simulink subsystem "PathFollowingController"  (R2022a)
settings: Solver=VariableStepAuto  StartTime=0.0  StopTime=10.0  RelTol=1e-3
undefined symbols (not defined in the file): constr, DE2019, DiscIntNeverNeededParam, ENVMT, Lbooth, loiterStates, params
libraries: simulink x16, dspsigops x1
(part 1 of 2)
settings Model: Creator=dylaneijkelhof  LastModifiedBy=kebl6571
settings SolverCC: AlgebraicLoopSolver=TrustRegion
settings DebuggingCC: UnconnectedInputMsg=warning  UnconnectedOutputMsg=warning  UnconnectedLineMsg=warning  SFMachineParentedDataDiag=warning

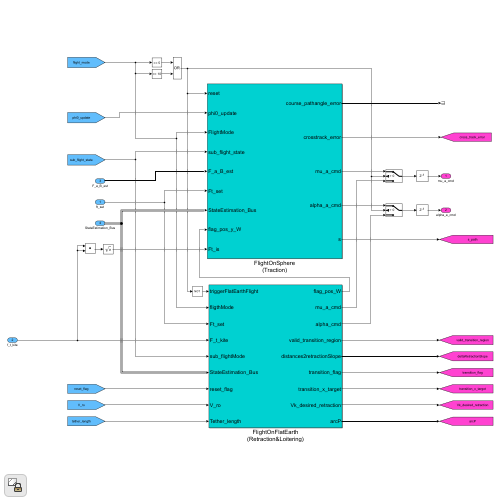
[thumbnail: Simulink's stored preview of the top-level diagram]
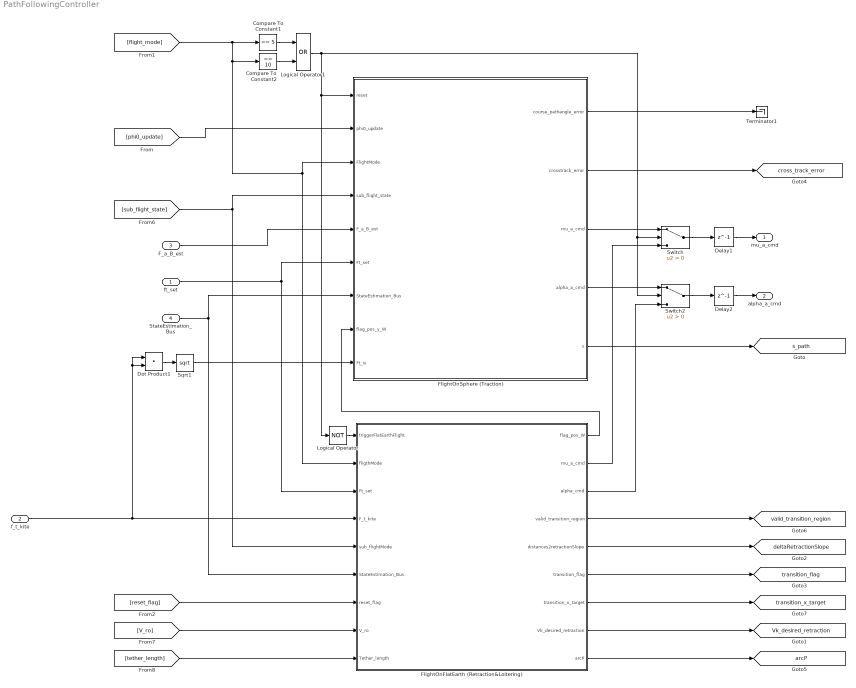
== system PathFollowingController ==
  ft_set : Inport
  f_t_kite : Inport  Port=2
  F_a_B_est : Inport  Port=3  PortDimensions=[3,1]
  StateEstimation_Bus : Inport  Port=4
  Compare To Constant1 : simulink/Logic and Bit Operations/Compare To Constant  relop===  const=5  OutDataTypeStr=boolean
  Compare To Constant2 : simulink/Logic and Bit Operations/Compare To Constant  relop===  const=10  OutDataTypeStr=boolean
  Delay1 : Delay  DelayLength=1
  Delay2 : Delay  DelayLength=1
  Dot Product1 : DotProduct  OutDataTypeStr=Inherit: Inherit via internal rule
  FlightOnFlatEarth (Retraction&Loitering) : Subsystem
  FlightOnSphere (Traction) : Subsystem
  Logical Operator : Logic  Operator=NOT  AllPortsSameDT=off  OutDataTypeStr=boolean
  Logical Operator1 : Logic  Operator=OR  AllPortsSameDT=off  OutDataTypeStr=boolean
  Sqrt1 : Sqrt
  Switch : Switch  Criteria=u2 > Threshold  SaturateOnIntegerOverflow=off  InputSameDT=off
  Switch2 : Switch  Criteria=u2 > Threshold  SaturateOnIntegerOverflow=off  InputSameDT=off
  Terminator1 : Terminator
  mu_a_cmd : Outport  PortDimensions=1  VectorParamsAs1DForOutWhenUnconnected=off
  alpha_a_cmd : Outport  Port=2  PortDimensions=1  VectorParamsAs1DForOutWhenUnconnected=off
  tag scope: Vk_desired_retraction=global, arcP=global, cross_track_error=global, deltaRetractionSlope=global, s_path=global, transition_flag=global, transition_x_target=global, valid_transition_region=global
  wires:
  StateEstimation_Bus/1 -> FlightOnSphere (Traction)/7(StateEstimation_Bus), FlightOnFlatEarth (Retraction&Loitering)/6(StateEstimation_Bus)
  Logical Operator1/1 -> FlightOnSphere (Traction)/1(reset), Logical Operator/1, Switch/2, Switch2/2
  FlightOnFlatEarth (Retraction&Loitering)/4(valid_transition_region) -> [valid_transition_region]
  FlightOnFlatEarth (Retraction&Loitering)/3(alpha_cmd) -> Switch2/3
  FlightOnFlatEarth (Retraction&Loitering)/2(mu_a_cmd) -> Switch/3
  Logical Operator/1 -> FlightOnFlatEarth (Retraction&Loitering)/1(triggerFlatEarthFlight)
  ft_set/1 -> FlightOnFlatEarth (Retraction&Loitering)/3(Ft_set), FlightOnSphere (Traction)/6(Ft_set)
  Delay2/1 -> alpha_a_cmd/1
  Delay1/1 -> mu_a_cmd/1
  Switch/1 -> Delay1/1
  Switch2/1 -> Delay2/1
  f_t_kite/1 -> Dot Product1/2, Dot Product1/1, FlightOnFlatEarth (Retraction&Loitering)/4(F_t_kite)
  F_a_B_est/1 -> FlightOnSphere (Traction)/5(F_a_B_est)
  FlightOnSphere (Traction)/4(alpha_a_cmd) -> Switch2/1
  FlightOnSphere (Traction)/3(mu_a_cmd) -> Switch/1
  FlightOnSphere (Traction)/1(course_pathangle_error) -> Terminator1/1
  FlightOnSphere (Traction)/2(crosstrack_error) -> [cross_track_error]
  [flight_mode] -> Compare To Constant1/1, FlightOnFlatEarth (Retraction&Loitering)/2(fligthMode), FlightOnSphere (Traction)/3(FlightMode), Compare To Constant2/1
  Compare To Constant1/1 -> Logical Operator1/1
  Compare To Constant2/1 -> Logical Operator1/2
  FlightOnSphere (Traction)/5(s) -> [s_path]
  [phi0_update] -> FlightOnSphere (Traction)/2(phi0_update)
  FlightOnFlatEarth (Retraction&Loitering)/6(transition_flag) -> [transition_flag]
  [reset_flag] -> FlightOnFlatEarth (Retraction&Loitering)/7(reset_flag)
  FlightOnFlatEarth (Retraction&Loitering)/5(distances2retractionSlope) -> [deltaRetractionSlope]
  FlightOnFlatEarth (Retraction&Loitering)/1(flag_pos_W) -> FlightOnSphere (Traction)/8(flag_pos_y_W)
  FlightOnFlatEarth (Retraction&Loitering)/7(transition_x_target) -> [transition_x_target]
  FlightOnFlatEarth (Retraction&Loitering)/8(Vk_desired_retraction) -> [Vk_desired_retraction]
  [V_ro] -> FlightOnFlatEarth (Retraction&Loitering)/8(V_ro)
  [tether_length] -> FlightOnFlatEarth (Retraction&Loitering)/9(Tether_length)
  [sub_flight_state] -> FlightOnFlatEarth (Retraction&Loitering)/5(sub_flightMode), FlightOnSphere (Traction)/4(sub_flight_state)
  FlightOnFlatEarth (Retraction&Loitering)/9(arcP) -> [arcP]
  Sqrt1/1 -> FlightOnSphere (Traction)/9(Ft_is)
  Dot Product1/1 -> Sqrt1/1

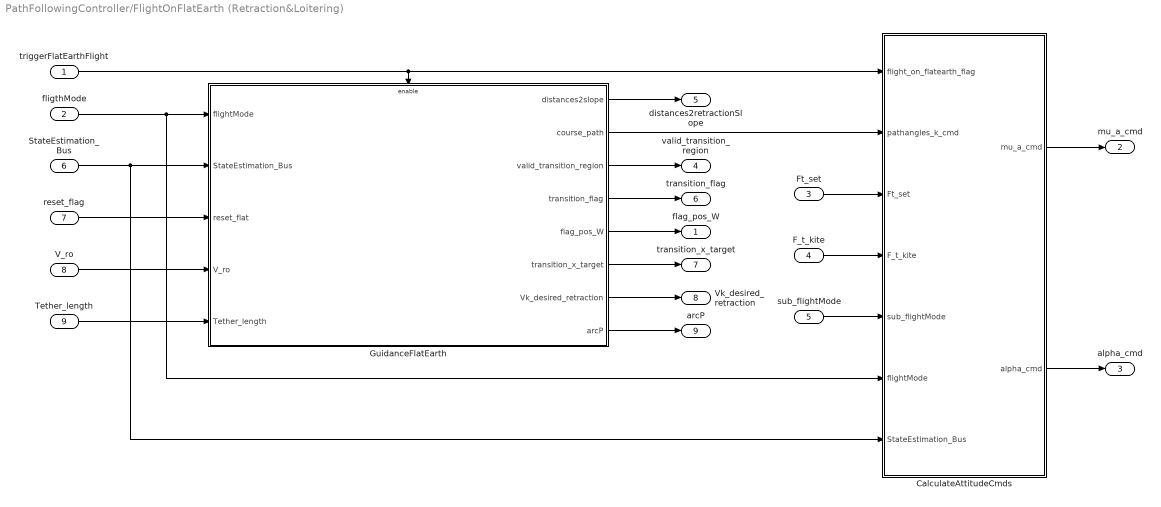
== system PathFollowingController/FlightOnFlatEarth (Retraction&Loitering) ==
  triggerFlatEarthFlight : Inport
  fligthMode : Inport  Port=2
  Ft_set : Inport  Port=3
  F_t_kite : Inport  Port=4
  sub_flightMode : Inport  Port=5
  StateEstimation_Bus : Inport  Port=6
  reset_flag : Inport  Port=7
  V_ro : Inport  Port=8
  Tether_length : Inport  Port=9
  CalculateAttitudeCmds : Subsystem
  GuidanceFlatEarth : Subsystem
  flag_pos_W : Outport  VectorParamsAs1DForOutWhenUnconnected=off
  mu_a_cmd : Outport  Port=2  VectorParamsAs1DForOutWhenUnconnected=off
  alpha_cmd : Outport  Port=3  VectorParamsAs1DForOutWhenUnconnected=off
  valid_transition_region : Outport  Port=4  VectorParamsAs1DForOutWhenUnconnected=off
  distances2retractionSlope : Outport  Port=5  VectorParamsAs1DForOutWhenUnconnected=off
  transition_flag : Outport  Port=6  VectorParamsAs1DForOutWhenUnconnected=off
  transition_x_target : Outport  Port=7  VectorParamsAs1DForOutWhenUnconnected=off
  Vk_desired_retraction : Outport  Port=8  VectorParamsAs1DForOutWhenUnconnected=off
  arcP : Outport  Port=9  VectorParamsAs1DForOutWhenUnconnected=off
  wires:
  GuidanceFlatEarth/8(arcP) -> arcP/1
  Tether_length/1 -> GuidanceFlatEarth/5(Tether_length)
  V_ro/1 -> GuidanceFlatEarth/4(V_ro)
  GuidanceFlatEarth/7(Vk_desired_retraction) -> Vk_desired_retraction/1
  GuidanceFlatEarth/6(transition_x_target) -> transition_x_target/1
  GuidanceFlatEarth/5(flag_pos_W) -> flag_pos_W/1
  reset_flag/1 -> GuidanceFlatEarth/3(reset_flat)
  GuidanceFlatEarth/4(transition_flag) -> transition_flag/1
  sub_flightMode/1 -> CalculateAttitudeCmds/5(sub_flightMode)
  GuidanceFlatEarth/2(course_path) -> CalculateAttitudeCmds/2(pathangles_k_cmd)
  GuidanceFlatEarth/1(distances2slope) -> distances2retractionSlope/1
  F_t_kite/1 -> CalculateAttitudeCmds/4(F_t_kite)
  GuidanceFlatEarth/3(valid_transition_region) -> valid_transition_region/1
  triggerFlatEarthFlight/1 -> CalculateAttitudeCmds/1(flight_on_flatearth_flag), GuidanceFlatEarth/Enable
  fligthMode/1 -> GuidanceFlatEarth/1(flightMode), CalculateAttitudeCmds/6(flightMode)
  CalculateAttitudeCmds/2(alpha_cmd) -> alpha_cmd/1
  Ft_set/1 -> CalculateAttitudeCmds/3(Ft_set)
  CalculateAttitudeCmds/1(mu_a_cmd) -> mu_a_cmd/1
  StateEstimation_Bus/1 -> GuidanceFlatEarth/2(StateEstimation_Bus), CalculateAttitudeCmds/7(StateEstimation_Bus)

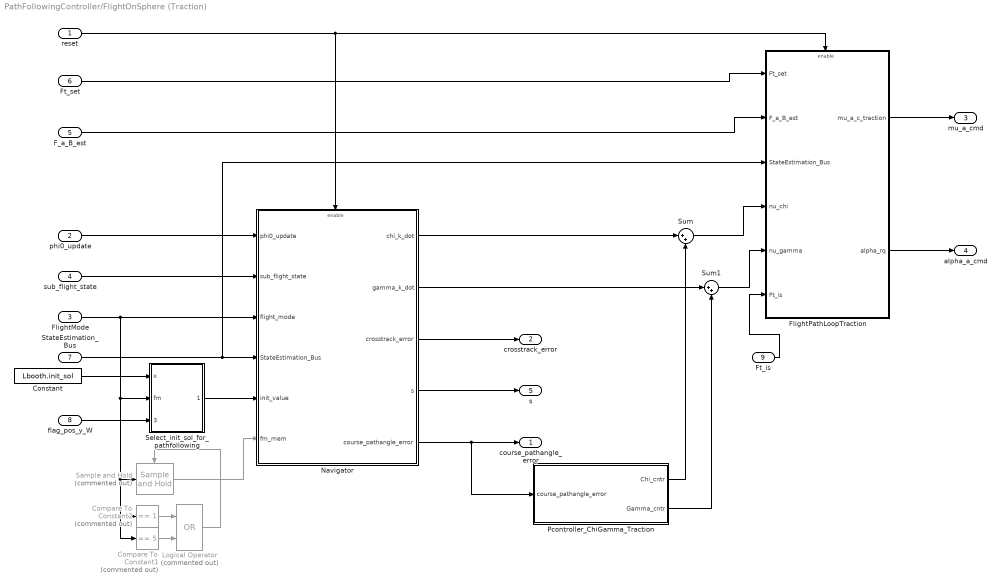
== system PathFollowingController/FlightOnSphere (Traction) ==
  reset : Inport
  phi0_update : Inport  Port=2
  FlightMode : Inport  Port=3  PortDimensions=1
  sub_flight_state : Inport  Port=4
  F_a_B_est : Inport  Port=5  PortDimensions=[3,1]
  Ft_set : Inport  Port=6
  StateEstimation_Bus : Inport  Port=7
  flag_pos_y_W : Inport  Port=8
  Ft_is : Inport  Port=9
  Compare To Constant1 : simulink/Logic and Bit Operations/Compare To Constant  Commented=on  relop===  const=5  OutDataTypeStr=boolean
  Compare To Constant2 : simulink/Logic and Bit Operations/Compare To Constant  Commented=on  relop===  const=1  OutDataTypeStr=boolean
  Constant : Constant  Value=Lbooth.init_sol
  FlightPathLoopTraction : Subsystem
  Logical Operator : Logic  Commented=on  Operator=OR  AllPortsSameDT=off  OutDataTypeStr=boolean
  Navigator : Subsystem
  Pcontroller_ChiGamma_Traction : Subsystem
  Sample and Hold : dspsigops/Sample and Hold  Commented=on  trig=Rising edge  initCond=0  latchinput=off
  Select_init_sol_for_pathfollowing : Stateflow chart  TreatAsAtomicUnit=on
  Sum : Sum  Inputs=|++
  Sum1 : Sum  Inputs=|++
  course_pathangle_error : Outport  VectorParamsAs1DForOutWhenUnconnected=off
  crosstrack_error : Outport  Port=2  VectorParamsAs1DForOutWhenUnconnected=off
  mu_a_cmd : Outport  Port=3  PortDimensions=1  VectorParamsAs1DForOutWhenUnconnected=off
  alpha_a_cmd : Outport  Port=4  PortDimensions=1  VectorParamsAs1DForOutWhenUnconnected=off
  s : Outport  Port=5  VectorParamsAs1DForOutWhenUnconnected=off
  wires:
  Ft_is/1 -> FlightPathLoopTraction/6(Ft_is)
  sub_flight_state/1 -> Navigator/2(sub_flight_state)
  Sample and Hold/1 -> Navigator/6(fm_mem)
  Logical Operator/1 -> Sample and Hold/Trigger
  Compare To Constant1/1 -> Logical Operator/2
  Compare To Constant2/1 -> Logical Operator/1
  Pcontroller_ChiGamma_Traction/2(Gamma_cntr) -> Sum1/2
  Pcontroller_ChiGamma_Traction/1(Chi_cntr) -> Sum/2
  flag_pos_y_W/1 -> Select_init_sol_for_pathfollowing/3(flag_pos_y_W)
  FlightMode/1 -> Select_init_sol_for_pathfollowing/2(fm), Compare To Constant1/1, Compare To Constant2/1, Sample and Hold/1, Navigator/3(flight_mode)
  Sum/1 -> FlightPathLoopTraction/4(nu_chi)
  Sum1/1 -> FlightPathLoopTraction/5(nu_gamma)
  Constant/1 -> Select_init_sol_for_pathfollowing/1(x)
  Select_init_sol_for_pathfollowing/1(sol_init) -> Navigator/5(init_value)
  Navigator/2(gamma_k_dot) -> Sum1/1
  Navigator/1(chi_k_dot) -> Sum/1
  reset/1 -> FlightPathLoopTraction/Enable, Navigator/Enable
  phi0_update/1 -> Navigator/1(phi0_update)
  Navigator/4(s) -> s/1
  StateEstimation_Bus/1 -> Navigator/4(StateEstimation_Bus), FlightPathLoopTraction/3(StateEstimation_Bus)
  Ft_set/1 -> FlightPathLoopTraction/1(Ft_set)
  F_a_B_est/1 -> FlightPathLoopTraction/2(F_a_B_est)
  FlightPathLoopTraction/2(alpha_rq) -> alpha_a_cmd/1
  Navigator/3(crosstrack_error) -> crosstrack_error/1
  Navigator/5(course_pathangle_error) -> course_pathangle_error/1, Pcontroller_ChiGamma_Traction/1(course_pathangle_error)
  FlightPathLoopTraction/1(mu_a_c_traction) -> mu_a_cmd/1

== system PathFollowingController/FlightOnFlatEarth (Retraction&Loitering)/CalculateAttitudeCmds ==
  flight_on_flatearth_flag : Inport
  pathangles_k_cmd : Inport  Port=2
  Ft_set : Inport  Port=3
  F_t_kite : Inport  Port=4
  sub_flightMode : Inport  Port=5
  flightMode : Inport  Port=6
  StateEstimation_Bus : Inport  Port=7
  Demux : Demux  Outputs=3
  FlightPathLoopRetraction_Aerodynamic : Subsystem
  Mux1 : Mux  Inputs=3
  Signal Specification : SignalSpecification  Dimensions=[3,1]
  Terminator2 : Terminator
  mu_a_cmd : Outport  VectorParamsAs1DForOutWhenUnconnected=off
  alpha_cmd : Outport  Port=2  VectorParamsAs1DForOutWhenUnconnected=off
  wires:
  sub_flightMode/1 -> FlightPathLoopRetraction_Aerodynamic/6(sub_flightMode)
  pathangles_k_cmd/1 -> FlightPathLoopRetraction_Aerodynamic/5(kinematic_path_cmd)
  FlightPathLoopRetraction_Aerodynamic/3(beta_a_cmd) -> Mux1/3
  Ft_set/1 -> FlightPathLoopRetraction_Aerodynamic/2(F_t_set)
  FlightPathLoopRetraction_Aerodynamic/1(mu_a_cmd) -> Mux1/1
  F_t_kite/1 -> FlightPathLoopRetraction_Aerodynamic/3(F_t_kite)
  Mux1/1 -> Signal Specification/1
  Demux/1 -> mu_a_cmd/1
  Signal Specification/1 -> Demux/1
  flightMode/1 -> FlightPathLoopRetraction_Aerodynamic/1(flight_mode)
  FlightPathLoopRetraction_Aerodynamic/2(alpha_a_cmd) -> Mux1/2
  flight_on_flatearth_flag/1 -> FlightPathLoopRetraction_Aerodynamic/Enable
  Demux/2 -> alpha_cmd/1
  Demux/3 -> Terminator2/1
  StateEstimation_Bus/1 -> FlightPathLoopRetraction_Aerodynamic/4(StateEstimation_Bus)

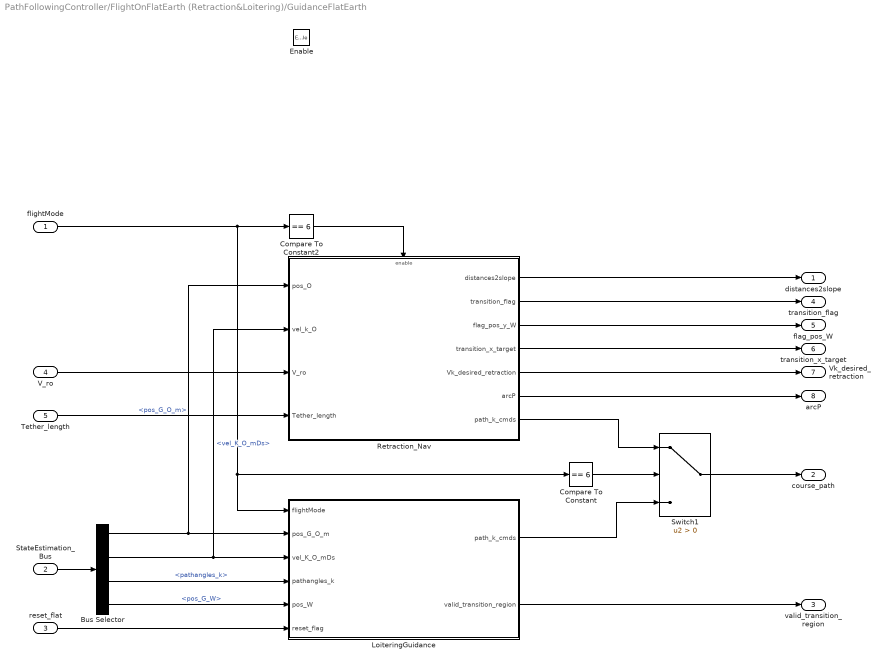
== system PathFollowingController/FlightOnFlatEarth (Retraction&Loitering)/GuidanceFlatEarth ==
  flightMode : Inport
  StateEstimation_Bus : Inport  Port=2
  reset_flat : Inport  Port=3
  V_ro : Inport  Port=4
  Tether_length : Inport  Port=5
  Enable : EnablePort
  Bus Selector : BusSelector  OutputSignals=pos_G_O_m,vel_K_O_mDs,pathangles_k,pos_G_W
  Compare To Constant : simulink/Logic and Bit Operations/Compare To Constant  relop===  const=6  OutDataTypeStr=boolean
  Compare To Constant2 : simulink/Logic and Bit Operations/Compare To Constant  relop===  const=6  OutDataTypeStr=boolean
  LoiteringGuidance : Subsystem
  Retraction_Nav : Subsystem
  Switch1 : Switch  Criteria=u2 > Threshold  SaturateOnIntegerOverflow=off  InputSameDT=off
  distances2slope : Outport  VectorParamsAs1DForOutWhenUnconnected=off
  course_path : Outport  Port=2  VectorParamsAs1DForOutWhenUnconnected=off
  valid_transition_region : Outport  Port=3  VectorParamsAs1DForOutWhenUnconnected=off
  transition_flag : Outport  Port=4  VectorParamsAs1DForOutWhenUnconnected=off
  flag_pos_W : Outport  Port=5  VectorParamsAs1DForOutWhenUnconnected=off
  transition_x_target : Outport  Port=6  VectorParamsAs1DForOutWhenUnconnected=off
  Vk_desired_retraction : Outport  Port=7  VectorParamsAs1DForOutWhenUnconnected=off
  arcP : Outport  Port=8  VectorParamsAs1DForOutWhenUnconnected=off
  wires:
  Retraction_Nav/6(arcP) -> arcP/1
  Tether_length/1 -> Retraction_Nav/4(Tether_length)
  V_ro/1 -> Retraction_Nav/3(V_ro)
  Retraction_Nav/5(Vk_desired_retraction) -> Vk_desired_retraction/1
  Retraction_Nav/4(transition_x_target) -> transition_x_target/1
  Retraction_Nav/3(flag_pos_y_W) -> flag_pos_W/1
  Bus Selector/4 -> LoiteringGuidance/5(pos_W)  "<pos_G_W>"
  reset_flat/1 -> LoiteringGuidance/6(reset_flag)
  Retraction_Nav/2(transition_flag) -> transition_flag/1
  LoiteringGuidance/2(valid_transition_region) -> valid_transition_region/1
  LoiteringGuidance/1(path_k_cmds) -> Switch1/3
  Bus Selector/3 -> LoiteringGuidance/4(pathangles_k)  "<pathangles_k>"
  flightMode/1 -> Compare To Constant2/1, Compare To Constant/1, LoiteringGuidance/1(flightMode)
  Retraction_Nav/7(path_k_cmds) -> Switch1/1
  Retraction_Nav/1(distances2slope) -> distances2slope/1
  Compare To Constant/1 -> Switch1/2
  Switch1/1 -> course_path/1
  Compare To Constant2/1 -> Retraction_Nav/Enable
  Bus Selector/2 -> LoiteringGuidance/3(vel_K_O_mDs), Retraction_Nav/2(vel_k_O)  "<vel_K_O_mDs>"
  StateEstimation_Bus/1 -> Bus Selector/1
  Bus Selector/1 -> LoiteringGuidance/2(pos_G_O_m), Retraction_Nav/1(pos_O)  "<pos_G_O_m>"

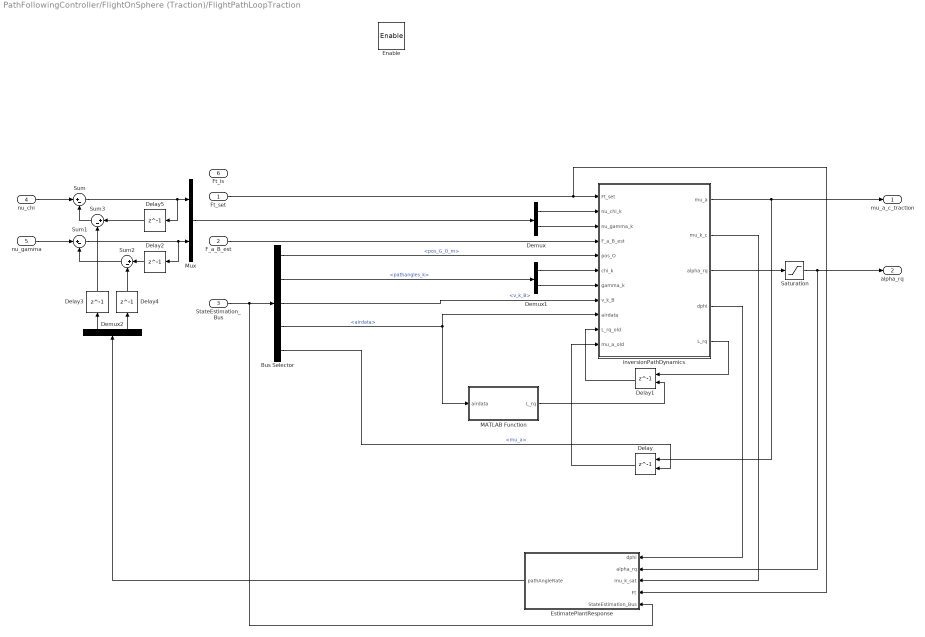
== system PathFollowingController/FlightOnSphere (Traction)/FlightPathLoopTraction ==
  Ft_set : Inport
  F_a_B_est : Inport  Port=2  PortDimensions=[3,1]
  StateEstimation_Bus : Inport  Port=3
  nu_chi : Inport  Port=4
  nu_gamma : Inport  Port=5
  Ft_is : Inport  Port=6
  Enable : EnablePort  StatesWhenEnabling=reset
  Bus Selector : BusSelector  OutputSignals=pos_G_O_m,pathangles_k,v_k_B,airdata,mu_a
  Delay : Delay  DelayLength=1  InitialConditionSource=Input port
      settings: InputPortMap=u0,p4
  Delay1 : Delay  DelayLength=1  InitialConditionSource=Input port
      settings: InputPortMap=u0,p4
  Delay{2..5} (4 alike) : Delay  DelayLength=1
  Demux : Demux  Outputs=2
  Demux1 : Demux  Outputs=2
  Demux2 : Demux  Outputs=2
  EstimatePlantResponse : Subsystem
  MATLAB Function : MATLAB Function  TreatAsAtomicUnit=on
  Mux : Mux  Inputs=2
  Saturation : Saturate  UpperLimit=constr.alpha_a_max  LowerLimit=constr.alpha_a_min
  Sum{,1..3} (4 alike) : Sum  Inputs=|+-
  inversionPathDynamics : MATLAB Function  TreatAsAtomicUnit=on
  mu_a_c_traction : Outport  PortDimensions=1  VectorParamsAs1DForOutWhenUnconnected=off
  alpha_rq : Outport  Port=2  PortDimensions=1  VectorParamsAs1DForOutWhenUnconnected=off
  wires:
  Ft_set/1 -> EstimatePlantResponse/4(Ft), inversionPathDynamics/1(Ft_set)
  Sum2/1 -> Sum1/2
  Demux2/1 -> Delay3/1
  nu_gamma/1 -> Sum1/1
  EstimatePlantResponse/1(pathAngleRate) -> Demux2/1
  Delay2/1 -> Sum2/1
  Sum/1 -> Delay5/1, Mux/1
  Sum1/1 -> Delay2/1, Mux/2
  Demux2/2 -> Delay4/1
  Delay3/1 -> Sum3/2
  Delay4/1 -> Sum2/2
  Sum3/1 -> Sum/2
  nu_chi/1 -> Sum/1
  Delay5/1 -> Sum3/1
  Bus Selector/1 -> inversionPathDynamics/5(pos_O)  "<pos_G_O_m>"
  Bus Selector/3 -> inversionPathDynamics/8(v_k_B)  "<v_k_B>"
  Bus Selector/2 -> Demux1/1  "<pathangles_k>"
  Bus Selector/4 -> MATLAB Function/1(airdata), inversionPathDynamics/9(airdata)  "<airdata>"
  StateEstimation_Bus/1 -> Bus Selector/1, EstimatePlantResponse/5(StateEstimation_Bus)
  Demux1/2 -> inversionPathDynamics/7(gamma_k)
  inversionPathDynamics/5(L_rq) -> Delay1/1
  MATLAB Function/1(L_rq) -> Delay1/2
  Delay/1 -> inversionPathDynamics/11(mu_a_old)
  Delay1/1 -> inversionPathDynamics/10(L_rq_old)
  inversionPathDynamics/4(dphi) -> EstimatePlantResponse/1(dphi)
  Saturation/1 -> EstimatePlantResponse/2(alpha_rq), alpha_rq/1
  inversionPathDynamics/3(alpha_rq) -> Saturation/1
  inversionPathDynamics/2(mu_k_c) -> EstimatePlantResponse/3(mu_k_sat)
  Demux/1 -> inversionPathDynamics/2(nu_chi_k)
  Demux/2 -> inversionPathDynamics/3(nu_gamma_k)
  Mux/1 -> Demux/1
  inversionPathDynamics/1(mu_a) -> mu_a_c_traction/1, Delay/1
  Demux1/1 -> inversionPathDynamics/6(chi_k)
  F_a_B_est/1 -> inversionPathDynamics/4(F_a_B_est)
  Bus Selector/5 -> Delay/2  "<mu_a>"

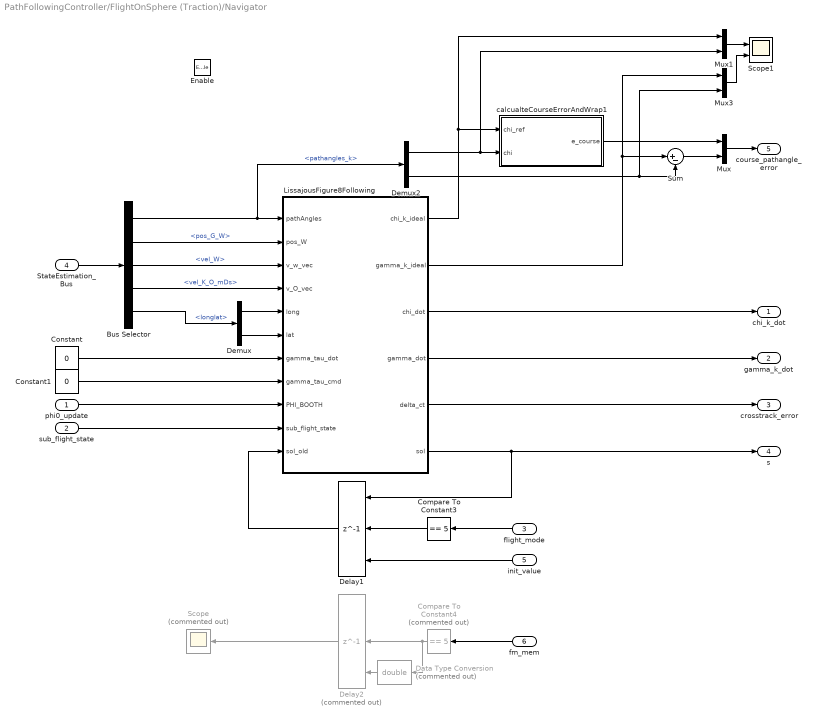
== system PathFollowingController/FlightOnSphere (Traction)/Navigator ==
  phi0_update : Inport
  sub_flight_state : Inport  Port=2
  flight_mode : Inport  Port=3
  StateEstimation_Bus : Inport  Port=4
  init_value : Inport  Port=5
  fm_mem : Inport  Port=6
  Enable : EnablePort  StatesWhenEnabling=reset
  Bus Selector : BusSelector  OutputSignals=pathangles_k,pos_G_W,vel_W,vel_K_O_mDs,longlat
  Compare To Constant3 : simulink/Logic and Bit Operations/Compare To Constant  relop===  const=5  OutDataTypeStr=boolean
  Compare To Constant4 : simulink/Logic and Bit Operations/Compare To Constant  Commented=on  relop===  const=5  OutDataTypeStr=boolean
  Constant : Constant  Value=0
  Constant1 : Constant  Value=0
  Data Type Conversion : DataTypeConversion  Commented=on  OutDataTypeStr=double  SaturateOnIntegerOverflow=off  RndMeth=Floor
  Delay1 : Delay  DelayLength=1  InitialConditionSource=Input port  InitialCondition=pi/2  ExternalReset=Rising
      settings: InputPortMap=u0,r5,p4
  Delay2 : Delay  Commented=on  DelayLength=1  InitialConditionSource=Input port  InitialCondition=pi/2  ExternalReset=Rising
      settings: InputPortMap=u0,r5,p4
  Demux : Demux  Outputs=2
  Demux2 : Demux  Outputs=2
  LissajousFigure8Following : MATLAB Function  TreatAsAtomicUnit=on
  Mux : Mux  Inputs=2
  Mux1 : Mux  Inputs=2
  Mux3 : Mux  Inputs=2
  Scope : Scope  Commented=on
  Scope1 : Scope  NumInputPorts=2
  Sum : Sum  Inputs=|+-
  calcualteCourseErrorAndWrap1 : MATLAB Function  TreatAsAtomicUnit=on
  chi_k_dot : Outport  PortDimensions=1  VectorParamsAs1DForOutWhenUnconnected=off
  gamma_k_dot : Outport  Port=2  PortDimensions=1  VectorParamsAs1DForOutWhenUnconnected=off
  crosstrack_error : Outport  Port=3  VectorParamsAs1DForOutWhenUnconnected=off
  s : Outport  Port=4  PortDimensions=1  InitialOutput=0  VectorParamsAs1DForOutWhenUnconnected=off
  course_pathangle_error : Outport  Port=5  VectorParamsAs1DForOutWhenUnconnected=off
  wires:
  sub_flight_state/1 -> LissajousFigure8Following/10(sub_flight_state)
  Data Type Conversion/1 -> Delay2/3
  fm_mem/1 -> Compare To Constant4/1
  Compare To Constant4/1 -> Data Type Conversion/1, Delay2/2
  Delay2/1 -> Scope/1
  Constant1/1 -> LissajousFigure8Following/8(gamma_tau_cmd)
  Bus Selector/3 -> LissajousFigure8Following/3(v_w_vec)  "<vel_W>"
  Constant/1 -> LissajousFigure8Following/7(gamma_tau_dot)
  init_value/1 -> Delay1/3
  Compare To Constant3/1 -> Delay1/2
  phi0_update/1 -> LissajousFigure8Following/9(PHI_BOOTH)
  flight_mode/1 -> Compare To Constant3/1
  Bus Selector/1 -> LissajousFigure8Following/1(pathAngles), Demux2/1  "<pathangles_k>"
  Bus Selector/5 -> Demux/1  "<longlat>"
  Bus Selector/2 -> LissajousFigure8Following/2(pos_W)  "<pos_G_W>"
  StateEstimation_Bus/1 -> Bus Selector/1
  LissajousFigure8Following/5(delta_ct) -> crosstrack_error/1
  Demux/2 -> LissajousFigure8Following/6(lat)
  Sum/1 -> Mux/2
  LissajousFigure8Following/3(chi_dot) -> chi_k_dot/1
  LissajousFigure8Following/4(gamma_dot) -> gamma_k_dot/1
  Mux/1 -> course_pathangle_error/1
  Demux2/2 -> Sum/2, Mux3/2
  Demux2/1 -> calcualteCourseErrorAndWrap1/2(chi), Mux1/2
  LissajousFigure8Following/2(gamma_k_ideal) -> Mux3/1, Sum/1
  LissajousFigure8Following/1(chi_k_ideal) -> Mux1/1, calcualteCourseErrorAndWrap1/1(chi_ref)
  calcualteCourseErrorAndWrap1/1(e_course) -> Mux/1
  Demux/1 -> LissajousFigure8Following/5(long)
  Bus Selector/4 -> LissajousFigure8Following/4(v_O_vec)  "<vel_K_O_mDs>"
  LissajousFigure8Following/6(sol) -> Delay1/1, s/1
  Delay1/1 -> LissajousFigure8Following/11(sol_old)
  Mux1/1 -> Scope1/1
  Mux3/1 -> Scope1/2

== system PathFollowingController/FlightOnSphere (Traction)/Pcontroller_ChiGamma_Traction ==
  course_pathangle_error : Inport
  Demux : Demux  Outputs=2
  Kp : Gain  Gain=params.Kp_gamma_k_traction  Multiplication=Matrix(K*u)
  Kp1 : Gain  Gain=params.Kp_chi_k_traction  Multiplication=Matrix(K*u)
  Chi_cntr : Outport
  Gamma_cntr : Outport  Port=2
  wires:
  Demux/1 -> Kp1/1
  Demux/2 -> Kp/1
  course_pathangle_error/1 -> Demux/1
  Kp/1 -> Gamma_cntr/1
  Kp1/1 -> Chi_cntr/1

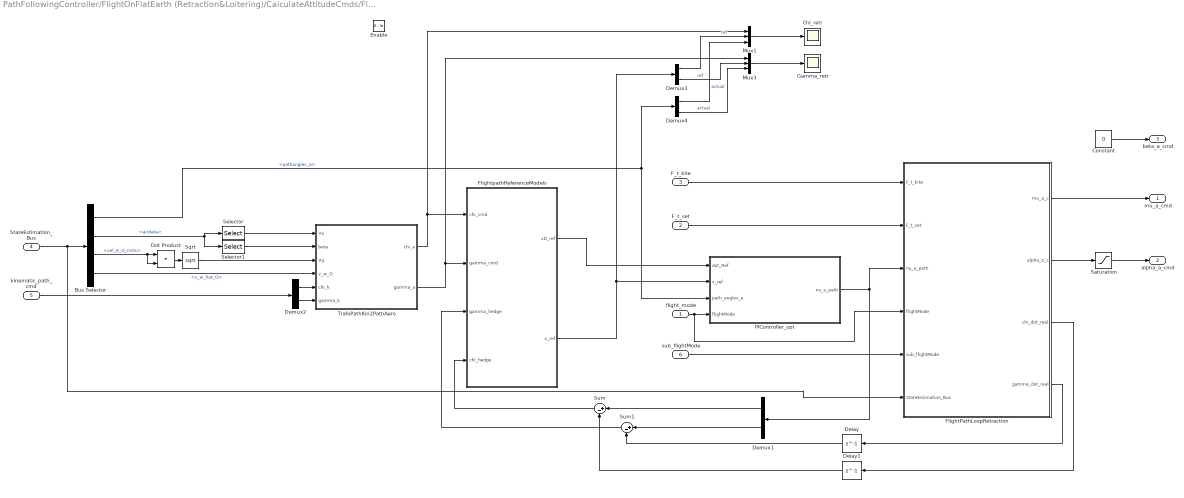
== system PathFollowingController/FlightOnFlatEarth (Retraction&Loitering)/CalculateAttitudeCmds/FlightPathLoopRetraction_Aerodynamic ==
  flight_mode : Inport
  F_t_set : Inport  Port=2
  F_t_kite : Inport  Port=3
  StateEstimation_Bus : Inport  Port=4
  kinematic_path_cmd : Inport  Port=5
  sub_flightMode : Inport  Port=6
  Enable : EnablePort  StatesWhenEnabling=reset
  Bus Selector : BusSelector  OutputSignals=pathangles_a,airdata,vel_K_O_mDs,v_w_hat_O
  Chi_retr : Scope
  Constant : Constant  Value=0
  Delay : Delay  DelayLength=1
  Delay1 : Delay  DelayLength=1
  Demux{1..4} (4 alike) : Demux  Outputs=2
  Dot Product : DotProduct  OutDataTypeStr=Inherit: Inherit via internal rule
  FlightPathLoopRetraction : Subsystem
  FlightpathReferenceModels : Subsystem
  Gamma_retr : Scope
  Mux1 : Mux  Inputs=3
  Mux3 : Mux  Inputs=3
  PIController_opt : Subsystem
  Saturation : Saturate  UpperLimit=constr.alpha_a_max  LowerLimit=constr.alpha_a_min
  Selector : Selector  InputPortWidth=3  IndexOptions=Index vector (dialog)  Indices=1  OutputSizes=1
  Selector1 : Selector  InputPortWidth=3  IndexOptions=Index vector (dialog)  Indices=3  OutputSizes=1
  Sqrt : Sqrt
  Sum : Sum  Inputs=|+-
  Sum1 : Sum  Inputs=|+-
  TrafoPathKin2PathAero : MATLAB Function  TreatAsAtomicUnit=on
  mu_a_cmd : Outport  VectorParamsAs1DForOutWhenUnconnected=off
  alpha_a_cmd : Outport  Port=2  VectorParamsAs1DForOutWhenUnconnected=off
  beta_a_cmd : Outport  Port=3  VectorParamsAs1DForOutWhenUnconnected=off
  wires:
  sub_flightMode/1 -> FlightPathLoopRetraction/5(sub_flightMode)
  Delay1/1 -> Sum/2
  Delay/1 -> Sum1/2
  Sum1/1 -> FlightpathReferenceModels/3(gamma_hedge)
  Sum/1 -> FlightpathReferenceModels/4(chi_hedge)
  Demux1/2 -> Sum1/1
  Demux1/1 -> Sum/1
  FlightPathLoopRetraction/4(gamma_dot_real) -> Delay/1
  flight_mode/1 -> FlightPathLoopRetraction/4(flightMode), PIController_opt/4(flightMode)
  Bus Selector/4 -> TrafoPathKin2PathAero/4(v_w_O)  "<v_w_hat_O>"
  kinematic_path_cmd/1 -> Demux2/1
  F_t_set/1 -> FlightPathLoopRetraction/2(F_t_set)
  Selector1/1 -> TrafoPathKin2PathAero/2(beta)
  TrafoPathKin2PathAero/2(gamma_a) -> FlightpathReferenceModels/2(gamma_cmd), Mux3/1
  TrafoPathKin2PathAero/1(chi_a) -> FlightpathReferenceModels/1(chi_cmd), Mux1/1
  Selector/1 -> TrafoPathKin2PathAero/1(Va)
  Sqrt/1 -> TrafoPathKin2PathAero/3(Vg)
  Dot Product/1 -> Sqrt/1
  FlightPathLoopRetraction/2(alpha_a_c) -> Saturation/1
  Saturation/1 -> alpha_a_cmd/1
  PIController_opt/1(nu_a_path) -> Demux1/1, FlightPathLoopRetraction/3(nu_a_path)
  FlightPathLoopRetraction/3(chi_dot_real) -> Delay1/1
  Constant/1 -> beta_a_cmd/1
  FlightpathReferenceModels/1(xD_ref) -> PIController_opt/1(dot_Ref)
  FlightPathLoopRetraction/1(mu_a_c) -> mu_a_cmd/1
  Demux2/1 -> TrafoPathKin2PathAero/5(chi_k)
  FlightpathReferenceModels/2(x_ref) -> PIController_opt/2(x_ref), Demux3/1
  Demux2/2 -> TrafoPathKin2PathAero/6(gamma_k)
  Demux3/1 -> Mux1/2  "ref"
  Demux4/2 -> Mux3/3  "actual"
  Demux3/2 -> Mux3/2  "ref"
  Demux4/1 -> Mux1/3  "actual"
  Mux1/1 -> Chi_retr/1
  Mux3/1 -> Gamma_retr/1
  F_t_kite/1 -> FlightPathLoopRetraction/1(F_t_kite)
  Bus Selector/2 -> Selector/1, Selector1/1  "<airdata>"
  Bus Selector/3 -> Dot Product/1, Dot Product/2  "<vel_K_O_mDs>"
  Bus Selector/1 -> PIController_opt/3(path_angles_a), Demux4/1  "<pathangles_a>"
  StateEstimation_Bus/1 -> FlightPathLoopRetraction/6(StateEstimation_Bus), Bus Selector/1

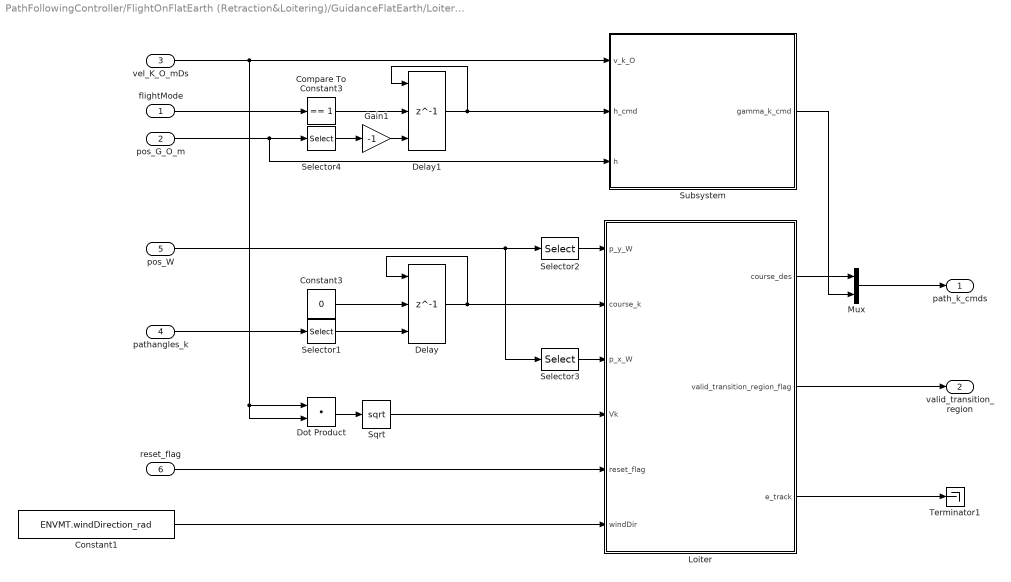
== system PathFollowingController/FlightOnFlatEarth (Retraction&Loitering)/GuidanceFlatEarth/LoiteringGuidance ==
  flightMode : Inport
  pos_G_O_m : Inport  Port=2
  vel_K_O_mDs : Inport  Port=3
  pathangles_k : Inport  Port=4
  pos_W : Inport  Port=5
  reset_flag : Inport  Port=6
  Compare To Constant3 : simulink/Logic and Bit Operations/Compare To Constant  relop===  const=1  OutDataTypeStr=boolean
  Constant1 : Constant  Value=ENVMT.windDirection_rad
  Constant3 : Constant  Value=0
  Delay : Delay  DelayLength=1  InitialConditionSource=Input port  ExternalReset=Rising
      settings: InputPortMap=u0,r5,p4
  Delay1 : Delay  DelayLength=1  InitialConditionSource=Input port  ExternalReset=Rising
      settings: InputPortMap=u0,r5,p4
  Dot Product : DotProduct  OutDataTypeStr=Inherit: Inherit via internal rule
  Gain1 : Gain  Gain=-1
  Loiter : Stateflow chart  TreatAsAtomicUnit=on  mask{kp_course_init=loiterStates.kp_delta_course, pos_OLoiter_W=loiterStates.pos_OLoiter_W, R_init_loiter=loiterStates.R, validTransReg_start=loiterStates.validTransReg_start, validTransReg_end=loiterStates.validTransReg_end}
  Mux : Mux  Inputs=2
  Selector1 : Selector  InputPortWidth=2  IndexOptions=Index vector (dialog)  Indices=1  OutputSizes=1
  Selector2 : Selector  InputPortWidth=3  IndexOptions=Index vector (dialog)  Indices=2  OutputSizes=1
  Selector3 : Selector  InputPortWidth=3  IndexOptions=Index vector (dialog)  Indices=1  OutputSizes=1
  Selector4 : Selector  InputPortWidth=3  IndexOptions=Index vector (dialog)  Indices=3  OutputSizes=1
  Sqrt : Sqrt
  Subsystem : Subsystem
  Terminator1 : Terminator
  path_k_cmds : Outport  VectorParamsAs1DForOutWhenUnconnected=off
  valid_transition_region : Outport  Port=2  VectorParamsAs1DForOutWhenUnconnected=off
  wires:
  Loiter/3(e_track) -> Terminator1/1
  flightMode/1 -> Compare To Constant3/1
  Constant3/1 -> Delay/2
  Constant1/1 -> Loiter/6(windDir)
  reset_flag/1 -> Loiter/5(reset_flag)
  Loiter/2(valid_transition_region_flag) -> valid_transition_region/1
  Selector2/1 -> Loiter/1(p_y_W)
  Delay/1 -> Delay/1, Loiter/2(course_k)
  Subsystem/1(gamma_k_cmd) -> Mux/2
  Gain1/1 -> Delay1/3
  Selector3/1 -> Loiter/3(p_x_W)
  pos_G_O_m/1 -> Selector4/1, Subsystem/3(h)
  vel_K_O_mDs/1 -> Dot Product/2, Dot Product/1, Subsystem/1(v_k_O)
  Loiter/1(course_des) -> Mux/1
  Delay1/1 -> Subsystem/2(h_cmd), Delay1/1
  Sqrt/1 -> Loiter/4(Vk)
  Dot Product/1 -> Sqrt/1
  pos_W/1 -> Selector3/1, Selector2/1
  Compare To Constant3/1 -> Delay1/2
  Selector4/1 -> Gain1/1
  Selector1/1 -> Delay/3
  Mux/1 -> path_k_cmds/1
  pathangles_k/1 -> Selector1/1

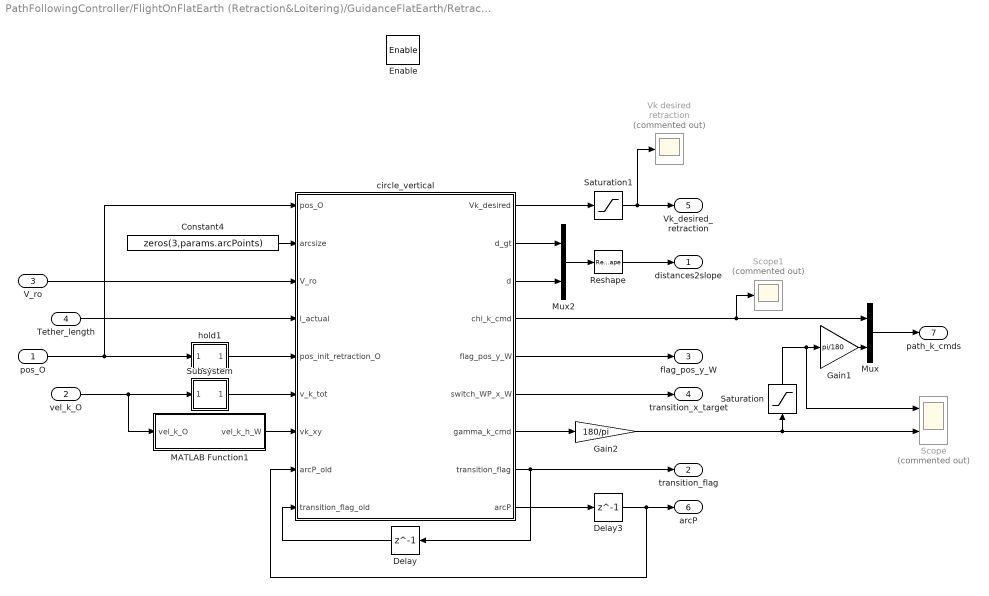
== system PathFollowingController/FlightOnFlatEarth (Retraction&Loitering)/GuidanceFlatEarth/Retraction_Nav ==
  pos_O : Inport
  vel_k_O : Inport  Port=2
  V_ro : Inport  Port=3
  Tether_length : Inport  Port=4
  Enable : EnablePort  StatesWhenEnabling=reset
  Constant4 : Constant  Value=zeros(3,params.arcPoints)
  Delay : Delay  DelayLength=1
  Delay3 : Delay  DelayLength=1  InitialCondition=zeros(3,params.arcPoints)
  Gain1 : Gain  Gain=pi/180
  Gain2 : Gain  Gain=180/pi
  MATLAB Function1 : MATLAB Function  TreatAsAtomicUnit=on
  Mux : Mux  Inputs=2
  Mux2 : Mux  Inputs=2
  Reshape : Reshape  OutputDimensionality=Row vector (2-D)
  Saturation : Saturate  UpperLimit=constr.gamma_max_retraction  LowerLimit=constr.gamma_min_retraction
  Saturation1 : Saturate  UpperLimit=300  LowerLimit=0
  Scope : Scope  Commented=on  NumInputPorts=2
  Scope1 : Scope  Commented=on
  Subsystem : Subsystem
      mask Display: disp('norm()')
  Vk desired retraction : Scope  Commented=on
  circle_vertical : MATLAB Function  TreatAsAtomicUnit=on
  hold1 : Subsystem
      mask Display: disp('hold()', 'texmode','on')
  distances2slope : Outport  VectorParamsAs1DForOutWhenUnconnected=off
  transition_flag : Outport  Port=2  VectorParamsAs1DForOutWhenUnconnected=off
  flag_pos_y_W : Outport  Port=3  VectorParamsAs1DForOutWhenUnconnected=off
  transition_x_target : Outport  Port=4  VectorParamsAs1DForOutWhenUnconnected=off
  Vk_desired_retraction : Outport  Port=5  VectorParamsAs1DForOutWhenUnconnected=off
  arcP : Outport  Port=6  VectorParamsAs1DForOutWhenUnconnected=off
  path_k_cmds : Outport  Port=7  PortDimensions=[2,1]  VectorParamsAs1DForOutWhenUnconnected=off
  wires:
  Subsystem/1(Out1) -> circle_vertical/6(v_k_tot)
  pos_O/1 -> hold1/1(In1), circle_vertical/1(pos_O)
  Delay3/1 -> arcP/1, circle_vertical/8(arcP_old)
  circle_vertical/9(arcP) -> Delay3/1
  Constant4/1 -> circle_vertical/2(arcsize)
  Saturation1/1 -> Vk_desired_retraction/1, Vk desired retraction/1
  circle_vertical/1(Vk_desired) -> Saturation1/1
  V_ro/1 -> circle_vertical/3(V_ro)
  Tether_length/1 -> circle_vertical/4(l_actual)
  Gain2/1 -> Scope/2, Saturation/1
  circle_vertical/6(switch_WP_x_W) -> transition_x_target/1
  circle_vertical/5(flag_pos_y_W) -> flag_pos_y_W/1
  Reshape/1 -> distances2slope/1
  Delay/1 -> circle_vertical/9(transition_flag_old)
  Mux/1 -> path_k_cmds/1
  Saturation/1 -> Scope/1, Gain1/1
  vel_k_O/1 -> MATLAB Function1/1(vel_k_O), Subsystem/1(In1)
  circle_vertical/3(d) -> Mux2/2
  hold1/1(Out1) -> circle_vertical/5(pos_init_retraction_O)
  Gain1/1 -> Mux/2
  circle_vertical/4(chi_k_cmd) -> Scope1/1, Mux/1
  Mux2/1 -> Reshape/1
  circle_vertical/2(d_gt) -> Mux2/1
  MATLAB Function1/1(vel_k_h_W) -> circle_vertical/7(vk_xy)
  circle_vertical/8(transition_flag) -> transition_flag/1, Delay/1
  circle_vertical/7(gamma_k_cmd) -> Gain2/1

== system PathFollowingController/FlightOnSphere (Traction)/FlightPathLoopTraction/EstimatePlantResponse ==
  dphi : Inport
  alpha_rq : Inport  Port=2
  mu_k_sat : Inport  Port=3
  Ft : Inport  Port=4
  StateEstimation_Bus : Inport  Port=5
  Bus Selector : BusSelector  OutputSignals=pathangles_k,pos_G_O_m,v_k_B,airdata
  Demux : Demux  Outputs=2
  MATLAB Function : MATLAB Function  TreatAsAtomicUnit=on
  Mux : Mux  Inputs=3
  Mux4 : Mux  Inputs=2
  Selector : Selector  InputPortWidth=3  IndexOptions=Index vector (dialog)  Indices=1  OutputSizes=1
  Selector1 : Selector  InputPortWidth=3  IndexOptions=Index vector (dialog)  Indices=3  OutputSizes=1
  pathAngleRate : Outport  VectorParamsAs1DForOutWhenUnconnected=off
  wires:
  Mux/1 -> MATLAB Function/8(airdata)
  alpha_rq/1 -> Mux/2
  Selector1/1 -> Mux/3
  Selector/1 -> Mux/1
  Bus Selector/1 -> Demux/1  "<pathangles_k>"
  Bus Selector/3 -> MATLAB Function/7(v_k_B)  "<v_k_B>"
  Bus Selector/4 -> Selector/1, Selector1/1  "<airdata>"
  Bus Selector/2 -> MATLAB Function/6(pos_O)  "<pos_G_O_m>"
  StateEstimation_Bus/1 -> Bus Selector/1
  mu_k_sat/1 -> MATLAB Function/3(mu_k)
  Ft/1 -> MATLAB Function/1(F_t)
  Demux/2 -> MATLAB Function/5(gamma_k)
  Demux/1 -> MATLAB Function/4(chi_k)
  dphi/1 -> MATLAB Function/2(dphi)
  MATLAB Function/1(chi_dot_real) -> Mux4/1
  Mux4/1 -> pathAngleRate/1
  MATLAB Function/2(gamma_dot_real) -> Mux4/2

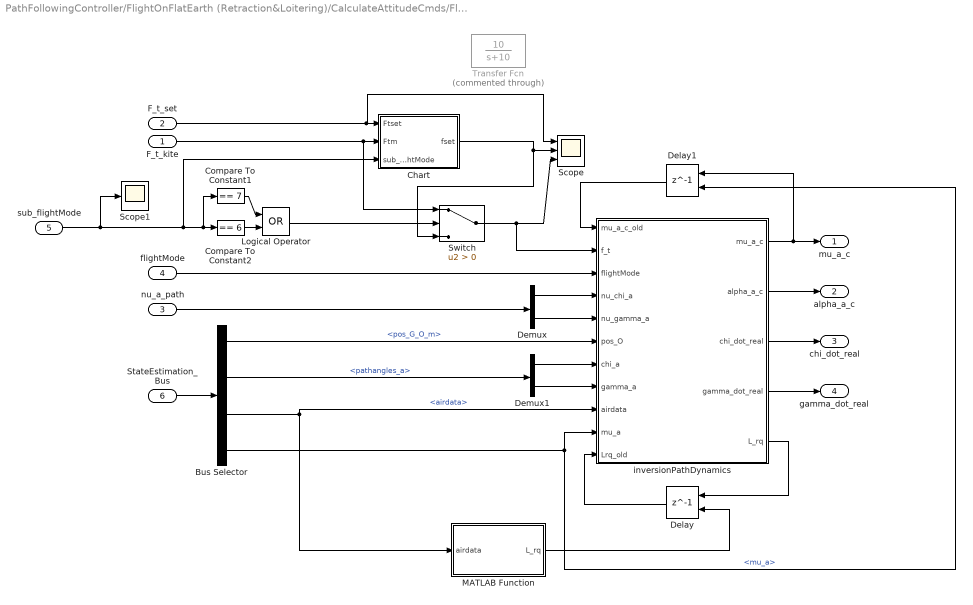
== system PathFollowingController/FlightOnFlatEarth (Retraction&Loitering)/CalculateAttitudeCmds/FlightPathLoopRetraction_Aerodynamic/FlightPathLoopRetraction ==
  F_t_kite : Inport
  F_t_set : Inport  Port=2
  nu_a_path : Inport  Port=3
  flightMode : Inport  Port=4
  sub_flightMode : Inport  Port=5
  StateEstimation_Bus : Inport  Port=6
  Bus Selector : BusSelector  OutputSignals=pos_G_O_m,pathangles_a,airdata,mu_a
  Chart : Stateflow chart  TreatAsAtomicUnit=on
  Compare To Constant1 : simulink/Logic and Bit Operations/Compare To Constant  relop===  const=7  OutDataTypeStr=boolean
  Compare To Constant2 : simulink/Logic and Bit Operations/Compare To Constant  relop===  const=6  OutDataTypeStr=boolean
  Delay : Delay  DelayLength=1  InitialConditionSource=Input port
      settings: InputPortMap=u0,p4
  Delay1 : Delay  DelayLength=1  InitialConditionSource=Input port
      settings: InputPortMap=u0,p4
  Demux : Demux  Outputs=2
  Demux1 : Demux  Outputs=2
  Logical Operator : Logic  Operator=OR  AllPortsSameDT=off  OutDataTypeStr=boolean
  MATLAB Function : MATLAB Function  TreatAsAtomicUnit=on
  Scope : Scope  NumInputPorts=3
  Scope1 : Scope
  Switch : Switch  Criteria=u2 > Threshold  SaturateOnIntegerOverflow=off  InputSameDT=off
  Transfer Fcn : TransferFcn  Commented=through  Numerator=[10]  Denominator=[1 10]
  inversionPathDynamics : MATLAB Function  TreatAsAtomicUnit=on
  mu_a_c : Outport  PortDimensions=1  VectorParamsAs1DForOutWhenUnconnected=off
  alpha_a_c : Outport  Port=2  PortDimensions=1  VectorParamsAs1DForOutWhenUnconnected=off
  chi_dot_real : Outport  Port=3  PortDimensions=1  VectorParamsAs1DForOutWhenUnconnected=off
  gamma_dot_real : Outport  Port=4  PortDimensions=1  VectorParamsAs1DForOutWhenUnconnected=off
  wires:
  Logical Operator/1 -> Switch/2
  Compare To Constant1/1 -> Logical Operator/1
  Compare To Constant2/1 -> Logical Operator/2
  sub_flightMode/1 -> Compare To Constant2/1, Compare To Constant1/1, Chart/3(sub_flightMode), Scope1/1
  Switch/1 -> inversionPathDynamics/2(f_t), Scope/3
  Chart/1(fset) -> Scope/2, Switch/3
  F_t_kite/1 -> Chart/2(Ftm), Switch/1
  F_t_set/1 -> Chart/1(Ftset), Scope/1
  inversionPathDynamics/4(gamma_dot_real) -> gamma_dot_real/1
  inversionPathDynamics/3(chi_dot_real) -> chi_dot_real/1
  inversionPathDynamics/5(L_rq) -> Delay/1
  Bus Selector/4 -> Delay1/2, inversionPathDynamics/10(mu_a)  "<mu_a>"
  Demux1/1 -> inversionPathDynamics/7(chi_a)
  inversionPathDynamics/2(alpha_a_c) -> alpha_a_c/1
  Demux/1 -> inversionPathDynamics/4(nu_chi_a)
  Demux/2 -> inversionPathDynamics/5(nu_gamma_a)
  nu_a_path/1 -> Demux/1
  flightMode/1 -> inversionPathDynamics/3(flightMode)
  Delay/1 -> inversionPathDynamics/11(Lrq_old)
  Delay1/1 -> inversionPathDynamics/1(mu_a_c_old)
  inversionPathDynamics/1(mu_a_c) -> mu_a_c/1, Delay1/1
  MATLAB Function/1(L_rq) -> Delay/2
  StateEstimation_Bus/1 -> Bus Selector/1
  Bus Selector/3 -> MATLAB Function/1(airdata), inversionPathDynamics/9(airdata)  "<airdata>"
  Bus Selector/2 -> Demux1/1  "<pathangles_a>"
  Demux1/2 -> inversionPathDynamics/8(gamma_a)
  Bus Selector/1 -> inversionPathDynamics/6(pos_O)  "<pos_G_O_m>"

== system PathFollowingController/FlightOnFlatEarth (Retraction&Loitering)/CalculateAttitudeCmds/FlightPathLoopRetraction_Aerodynamic/FlightpathReferenceModels ==
  chi_cmd : Inport
  gamma_cmd : Inport  Port=2
  gamma_hedge : Inport  Port=3
  chi_hedge : Inport  Port=4
  Mux2 : Mux  Inputs=2
  Mux3 : Mux  Inputs=2
  SecondOrderReferenceModel_course : Subsystem  mask{omega0_max=params.w0_chi_retraction_max, zeta0=1, y_max=inf, y_min=-inf, yd_max=inf, yd_min=-inf, y2d_max=inf, y2d_min=-inf}
  SecondOrderReferenceModel_pathangle : Subsystem  mask{omega0_max=params.w0_gamma_retraction_max, zeta0=1, y_max=inf, y_min=-inf, yd_max=inf, yd_min=-inf, y2d_max=inf, y2d_min=-inf}
  xD_ref : Outport  VectorParamsAs1DForOutWhenUnconnected=off
  x_ref : Outport  Port=2  VectorParamsAs1DForOutWhenUnconnected=off
  wires:
  SecondOrderReferenceModel_pathangle/2(y_ref_dot) -> Mux3/2
  SecondOrderReferenceModel_course/2(y_ref_dot) -> Mux3/1
  SecondOrderReferenceModel_pathangle/1(y_ref) -> Mux2/2
  SecondOrderReferenceModel_course/1(y_ref) -> Mux2/1
  Mux2/1 -> x_ref/1
  Mux3/1 -> xD_ref/1
  chi_cmd/1 -> SecondOrderReferenceModel_course/1(y_cmd)
  gamma_cmd/1 -> SecondOrderReferenceModel_pathangle/1(y_cmd)
  chi_hedge/1 -> SecondOrderReferenceModel_course/2(hedge)
  gamma_hedge/1 -> SecondOrderReferenceModel_pathangle/2(hedge)

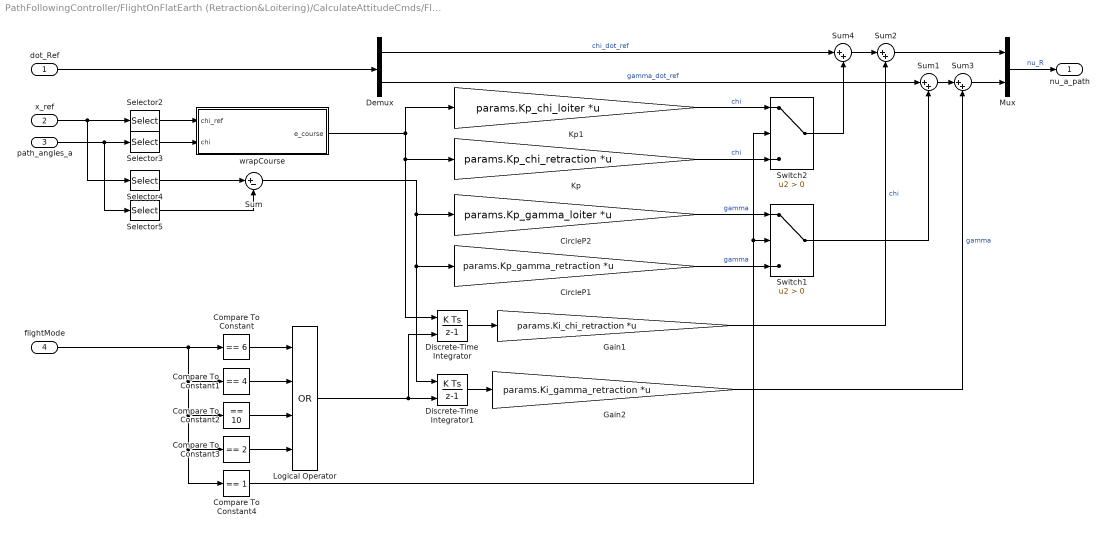
== system PathFollowingController/FlightOnFlatEarth (Retraction&Loitering)/CalculateAttitudeCmds/FlightPathLoopRetraction_Aerodynamic/PIController_opt ==
  dot_Ref : Inport
  x_ref : Inport  Port=2
  path_angles_a : Inport  Port=3
  flightMode : Inport  Port=4
  CircleP1 : Gain  Gain=params.Kp_gamma_retraction  Multiplication=Matrix(K*u)
  CircleP2 : Gain  Gain=params.Kp_gamma_loiter  Multiplication=Matrix(K*u)
  Compare To Constant : simulink/Logic and Bit Operations/Compare To Constant  relop===  const=6  OutDataTypeStr=boolean
  Compare To Constant1 : simulink/Logic and Bit Operations/Compare To Constant  relop===  const=4  OutDataTypeStr=boolean
  Compare To Constant2 : simulink/Logic and Bit Operations/Compare To Constant  relop===  const=10  OutDataTypeStr=boolean
  Compare To Constant3 : simulink/Logic and Bit Operations/Compare To Constant  relop===  const=2  OutDataTypeStr=boolean
  Compare To Constant4 : simulink/Logic and Bit Operations/Compare To Constant  relop===  const=1  OutDataTypeStr=boolean
  Demux : Demux  Outputs=2
  Discrete-Time Integrator : DiscreteIntegrator  ExternalReset=either  SampleTime=-1  ICPrevOutput=DiscIntNeverNeededParam  ICPrevScaledInput=DiscIntNeverNeededParam
  Discrete-Time Integrator1 : DiscreteIntegrator  ExternalReset=either  SampleTime=-1  ICPrevOutput=DiscIntNeverNeededParam  ICPrevScaledInput=DiscIntNeverNeededParam
  Gain1 : Gain  Gain=params.Ki_chi_retraction  Multiplication=Matrix(K*u) (u vector)
  Gain2 : Gain  Gain=params.Ki_gamma_retraction  Multiplication=Matrix(K*u) (u vector)
  Kp : Gain  Gain=params.Kp_chi_retraction  Multiplication=Matrix(K*u)
  Kp1 : Gain  Gain=params.Kp_chi_loiter  Multiplication=Matrix(K*u)
  Logical Operator : Logic  Operator=OR  Inputs=4  AllPortsSameDT=off  OutDataTypeStr=boolean
  Mux : Mux  Inputs=2
  Selector2 : Selector  InputPortWidth=2  IndexOptions=Index vector (dialog)  Indices=1  OutputSizes=1
  Selector3 : Selector  InputPortWidth=2  IndexOptions=Index vector (dialog)  Indices=1  OutputSizes=1
  Selector4 : Selector  InputPortWidth=2  IndexOptions=Index vector (dialog)  Indices=2  OutputSizes=1
  Selector5 : Selector  InputPortWidth=2  IndexOptions=Index vector (dialog)  Indices=2  OutputSizes=1
  Sum : Sum  Inputs=|+-
  Sum{1..4} (4 alike) : Sum  Inputs=|++
  Switch1 : Switch  Criteria=u2 > Threshold  SaturateOnIntegerOverflow=off  InputSameDT=off
  Switch2 : Switch  Criteria=u2 > Threshold  SaturateOnIntegerOverflow=off  InputSameDT=off
  wrapCourse : MATLAB Function  TreatAsAtomicUnit=on
  nu_a_path : Outport  VectorParamsAs1DForOutWhenUnconnected=off
  wires:
  Switch1/1 -> Sum1/2
  CircleP2/1 -> Switch1/1  "gamma"
  Kp1/1 -> Switch2/1  "chi"
  Switch2/1 -> Sum4/2
  Compare To Constant4/1 -> Switch1/2, Switch2/2
  Selector3/1 -> wrapCourse/2(chi)
  Selector5/1 -> Sum/2
  Sum3/1 -> Mux/2
  Sum2/1 -> Mux/1
  Discrete-Time Integrator/1 -> Gain1/1
  Gain2/1 -> Sum3/2  "gamma"
  Gain1/1 -> Sum2/2  "chi"
  x_ref/1 -> Selector2/1, Selector4/1
  Selector2/1 -> wrapCourse/1(chi_ref)
  Selector4/1 -> Sum/1
  path_angles_a/1 -> Selector3/1, Selector5/1
  Discrete-Time Integrator1/1 -> Gain2/1
  Compare To Constant2/1 -> Logical Operator/3
  Compare To Constant1/1 -> Logical Operator/2
  Compare To Constant/1 -> Logical Operator/1
  Sum/1 -> CircleP2/1, CircleP1/1, Discrete-Time Integrator1/1
  Sum1/1 -> Sum3/1
  CircleP1/1 -> Switch1/3  "gamma"
  Demux/2 -> Sum1/1  "gamma_dot_ref"
  wrapCourse/1(e_course) -> Kp1/1, Discrete-Time Integrator/1, Kp/1
  Sum4/1 -> Sum2/1
  Kp/1 -> Switch2/3  "chi"
  Demux/1 -> Sum4/1  "chi_dot_ref"
  dot_Ref/1 -> Demux/1
  Mux/1 -> nu_a_path/1  "nu_R"
  flightMode/1 -> Compare To Constant/1, Compare To Constant1/1, Compare To Constant3/1, Compare To Constant4/1, Compare To Constant2/1
  Logical Operator/1 -> Discrete-Time Integrator1/2, Discrete-Time Integrator/2
  Compare To Constant3/1 -> Logical Operator/4

== system PathFollowingController/FlightOnFlatEarth (Retraction&Loitering)/GuidanceFlatEarth/LoiteringGuidance/Subsystem ==
  v_k_O : Inport
  h_cmd : Inport  Port=2
  h : Inport  Port=3
  Asin : Trigonometry  Operator=asin
  Divide : Product  Inputs=*/
  Dot Product : DotProduct  OutDataTypeStr=Inherit: Inherit via internal rule
  Gain2 : Gain  Gain=-1
  Gain3 : Gain  Gain=loiterStates.kp_h
  Saturation : Saturate  UpperLimit=50*pi/180  LowerLimit=-50*pi/180
  Saturation1 : Saturate  UpperLimit=1  LowerLimit=-1
  Selector : Selector  InputPortWidth=3  IndexOptions=Index vector (dialog)  Indices=3  OutputSizes=1
  Sqrt : Sqrt
  Sum2 : Sum  Inputs=|-+
  gamma_k_cmd : Outport  VectorParamsAs1DForOutWhenUnconnected=off
  wires:
  Gain3/1 -> Divide/1
  Saturation1/1 -> Asin/1
  Asin/1 -> Saturation/1
  h/1 -> Selector/1
  v_k_O/1 -> Dot Product/2, Dot Product/1
  Dot Product/1 -> Sqrt/1
  Divide/1 -> Saturation1/1
  Sqrt/1 -> Divide/2
  Sum2/1 -> Gain3/1
  Gain2/1 -> Sum2/1
  Selector/1 -> Gain2/1
  Saturation/1 -> gamma_k_cmd/1
  h_cmd/1 -> Sum2/2

== system PathFollowingController/FlightOnFlatEarth (Retraction&Loitering)/GuidanceFlatEarth/Retraction_Nav/Subsystem ==
  In1 : Inport
  Dot Product3 : DotProduct  OutDataTypeStr=Inherit: Inherit via internal rule
  Sqrt1 : Sqrt
  Out1 : Outport
  wires:
  Dot Product3/1 -> Sqrt1/1
  Sqrt1/1 -> Out1/1
  In1/1 -> Dot Product3/2, Dot Product3/1

== system PathFollowingController/FlightOnFlatEarth (Retraction&Loitering)/GuidanceFlatEarth/Retraction_Nav/hold1 ==
  In1 : Inport
  Delay2 : Delay  DelayLength=1  InitialConditionSource=Input port  InitialCondition=zeros(3,1)
      settings: InputPortMap=u0,p4
  Out1 : Outport
  wires:
  Delay2/1 -> Delay2/1, Out1/1
  In1/1 -> Delay2/2

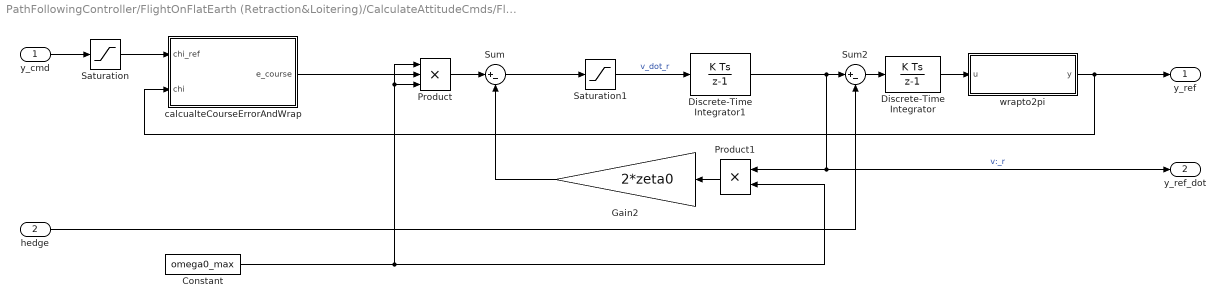
== system PathFollowingController/FlightOnFlatEarth (Retraction&Loitering)/CalculateAttitudeCmds/FlightPathLoopRetraction_Aerodynamic/FlightpathReferenceModels/SecondOrderReferenceModel_course ==
  y_cmd : Inport
  hedge : Inport  Port=2
  Constant : Constant  Value=omega0_max
  Discrete-Time Integrator : DiscreteIntegrator  SampleTime=-1  LimitOutput=on  UpperSaturationLimit=y_max  LowerSaturationLimit=y_min  ICPrevOutput=DiscIntNeverNeededParam  ICPrevScaledInput=DiscIntNeverNeededParam
  Discrete-Time Integrator1 : DiscreteIntegrator  SampleTime=-1  LimitOutput=on  UpperSaturationLimit=yd_max  LowerSaturationLimit=yd_min  ICPrevOutput=DiscIntNeverNeededParam  ICPrevScaledInput=DiscIntNeverNeededParam
  Gain2 : Gain  Gain=2*zeta0
  Product : Product  Inputs=3
  Product1 : Product
  Saturation : Saturate  UpperLimit=y_max  LowerLimit=y_min
  Saturation1 : Saturate  UpperLimit=y2d_max  LowerLimit=y2d_min
  Sum : Sum  Inputs=|+-
  Sum2 : Sum  Inputs=|+-
  calcualteCourseErrorAndWrap : MATLAB Function  TreatAsAtomicUnit=on
  wrapto2pi : MATLAB Function  TreatAsAtomicUnit=on
  y_ref : Outport  VectorParamsAs1DForOutWhenUnconnected=off
  y_ref_dot : Outport  Port=2  VectorParamsAs1DForOutWhenUnconnected=off
  wires:
  wrapto2pi/1(y) -> y_ref/1, calcualteCourseErrorAndWrap/2(chi)
  hedge/1 -> Sum2/2
  Sum2/1 -> Discrete-Time Integrator/1
  Saturation/1 -> calcualteCourseErrorAndWrap/1(chi_ref)
  Saturation1/1 -> Discrete-Time Integrator1/1  "v_dot_r"
  calcualteCourseErrorAndWrap/1(e_course) -> Product/2
  Gain2/1 -> Sum/2
  Sum/1 -> Saturation1/1
  Discrete-Time Integrator1/1 -> Sum2/1, Product1/1, y_ref_dot/1  "v:_r"
  y_cmd/1 -> Saturation/1
  Product/1 -> Sum/1
  Discrete-Time Integrator/1 -> wrapto2pi/1(u)
  Constant/1 -> Product/1, Product/3, Product1/2
  Product1/1 -> Gain2/1

== system PathFollowingController/FlightOnFlatEarth (Retraction&Loitering)/CalculateAttitudeCmds/FlightPathLoopRetraction_Aerodynamic/FlightpathReferenceModels/SecondOrderReferenceModel_pathangle ==
  y_cmd : Inport
  hedge : Inport  Port=2
  Constant : Constant  Value=omega0_max
  Discrete-Time Integrator : DiscreteIntegrator  SampleTime=-1  LimitOutput=on  UpperSaturationLimit=y_max  LowerSaturationLimit=y_min  ICPrevOutput=DiscIntNeverNeededParam  ICPrevScaledInput=DiscIntNeverNeededParam
  Discrete-Time Integrator1 : DiscreteIntegrator  SampleTime=-1  LimitOutput=on  UpperSaturationLimit=yd_max  LowerSaturationLimit=yd_min  ICPrevOutput=DiscIntNeverNeededParam  ICPrevScaledInput=DiscIntNeverNeededParam
  Gain2 : Gain  Gain=2*zeta0
  Product : Product  Inputs=3
  Product1 : Product
  Saturation : Saturate  UpperLimit=y_max  LowerLimit=y_min
  Saturation1 : Saturate  UpperLimit=y2d_max  LowerLimit=y2d_min
  Sum : Sum  Inputs=|+-
  Sum1 : Sum  Inputs=|+-
  Sum2 : Sum  Inputs=|+-
  y_ref : Outport  VectorParamsAs1DForOutWhenUnconnected=off
  y_ref_dot : Outport  Port=2  VectorParamsAs1DForOutWhenUnconnected=off
  wires:
  Discrete-Time Integrator/1 -> Sum1/2, y_ref/1
  hedge/1 -> Sum2/2
  Sum2/1 -> Discrete-Time Integrator/1
  Saturation/1 -> Sum1/1
  Saturation1/1 -> Discrete-Time Integrator1/1  "v_dot_r"
  Sum1/1 -> Product/2
  Gain2/1 -> Sum/2
  Sum/1 -> Saturation1/1
  Discrete-Time Integrator1/1 -> Sum2/1, Product1/1, y_ref_dot/1  "v:_r"
  y_cmd/1 -> Saturation/1
  Product/1 -> Sum/1
  Constant/1 -> Product/1, Product/3, Product1/2
  Product1/1 -> Gain2/1

== matlab function PathFollowingController/FlightOnFlatEarth (Retraction&Loitering)/CalculateAttitudeCmds/FlightPathLoopRetraction_Aerodynamic/FlightPathLoopRetraction/MATLAB Function ==
  data: L_rq output; airdata input; DE2019 parameter; constr parameter; ENVMT parameter
% Copyright 2021 Delft University of Technology
%
% Licensed under the Apache License, Version 2.0 (the "License");
% you may not use this file except in compliance with the License.
% You may obtain a copy of the License at
%
%      http://www.apache.org/licenses/LICENSE-2.0
%
% Unless required by applicable law or agreed to in writing, software
% distributed under the License is distributed on an "AS IS" BASIS,
% WITHOUT WARRANTIES OR CONDITIONS OF ANY KIND, either express or implied.
% See the License for the specific language governing permissions and
% limitations under the License.

function L_rq = fcn(airdata, DE2019,constr, ENVMT)
%fcn - Calculate required lift force
%
% Inputs:
%    airdata     - Airspeed, aoa, sideslip angle
%    DE2019     - Aircraft characteristics
%    constr     - Constraint, maximum lift
%
% Outputs:
%    L_rq    - Required lift
%
% Author: Sebastian Rapp, Ph.D., Revised by: Dylan Eijkelhof, M.Sc.
% Delft University of Technology
% email address: s.rapp@tudelft.nl
% email address: d.eijkelhof@tudelft.nl
% December 2019; Last revision: 06-October-2020

%-------------	BEGIN CODE	--------------

L_rq =  min( 0.5*ENVMT.rhos*DE2019.S_wing*airdata(1)^2 * (DE2019.CL0+DE2019.CL_alpha*airdata(2) ),constr.F_T_max); % max. negative lift

%-------------	 END CODE	--------------
end

== stateflow chart PathFollowingController/FlightOnFlatEarth (Retraction&Loitering)/CalculateAttitudeCmds/FlightPathLoopRetraction_Aerodynamic/FlightPathLoopRetraction/Chart ==
  settings: updateMethod=DISCRETE  sampleTime=0.1
  state ReducedSetforce
    during: fset = 0 ;
    during: t = t + 1;
  state Setforce
    during: fset = Ftset;
    entry: t=0;
  Setforce -> ReducedSetforce [commented out] : [Ftm>Ftset+1000]
  (default) -> Setforce
  Setforce -> ReducedSetforce : [sub_flightMode==6 || sub_flightMode == 7]
  ReducedSetforce -> Setforce : [sub_flightMode==8]
  ReducedSetforce -> Setforce [commented out] : [Ftm<Ftset-1000]
  data: Ftset input; Ftm input; fset output; t local; sub_flightMode input
